simulink model "LQR_simulink"  (Simulink 7.3)
settings: Solver=ode3  StartTime=0.0  StopTime=3  FixedStep=T  RelTol=1e-3
values from neighbouring files (symbols this model uses):
  A = [0 0 0 -85.6760374833 -12.5123773517 0 0 0 0 0 -18.6077643909 -80.8140678729 ... (49 elements, 7x7)]    [A.mat]    (also in CASEfinder.m = [0 1 0; -K/m -C/m 1/m;0 0 -1/tau]; Example_check_mLyapunov.m = [0 1 0; -K/m -C/m 1/m;0 0 -1/tau]; Example_check_mriccati.m = [0 1 0; -K/m -C/m 1/m;0 0 -1/tau]; Example_in_Kang_paper.m = A_actuator)
  B = [0 0 0 0 0 62.8318530718 0 0 0 0 0 0 ... (14 elements, 7x2)]    [B.mat]    (also in CASEfinder.m = [0;0;1/tau]; Example_check_mLyapunov.m = [0;0;1/tau]; Example_check_mriccati.m = [0;0;1/tau]; Example_in_Kang_paper.m = B_actuator)
  xf = [0;0;0]    [CASEfinder.m]    (also in Main_for_DOCandDODR.m = xfn; loopsimulation.m = xf_actuator)
  xi = [0;0;0]    [CASEfinder.m]    (also in Example_check_mLyapunov.m; Example_check_mriccati.m; Main_for_DOCandDODR.m = xin; StochasticRegulator.m = zeros(7,1))
undefined symbols (not defined in the file or in its folder): Kc, T
settings Model: Creator=JSPark  LastModifiedBy=JSPark

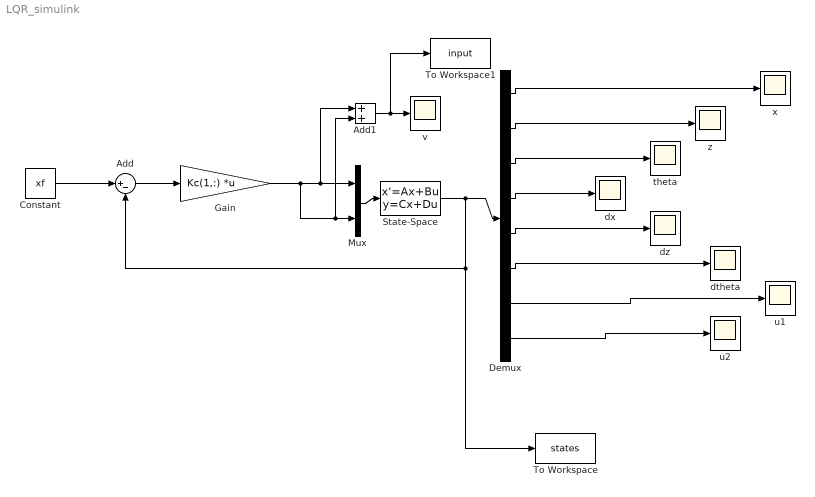
== system LQR_simulink ==
  Add : Sum  Inputs=|+-  OutDataType=fixdt(1, 16)  OutScaling=2^-10  SampleTime=T
  Add1 : Sum  OutDataType=fixdt(1, 16)  OutScaling=2^-10  SampleTime=T
  Constant : Constant  Value=xf  OutDataType=fixdt(1, 16)  OutScaling=2^0  SampleTime=T
  Demux : Demux  Outputs=8
  Gain : Gain  Gain=Kc(1,:)  Multiplication=Matrix(K*u)  ParameterDataType=fixdt(1, 16)  ParameterScaling=2^0  OutDataType=fixdt(1, 16)  OutScaling=2^0  SampleTime=T
  Mux : Mux  Inputs=2
  State-Space : StateSpace  A=A  B=B  C=eye(length(A))  D=zeros(length(A),2)  X0=xi
  To Workspace : ToWorkspace  VariableName=states  SampleTime=T  SaveFormat=Structure
  To Workspace1 : ToWorkspace  VariableName=input  SampleTime=T  SaveFormat=Structure
  dtheta : Scope
      settings: SaveName=ScopeData5
  dx : Scope
      settings: SaveName=ScopeData3
  dz : Scope
      settings: SaveName=ScopeData4
  theta : Scope
      settings: TimeRange=3  SaveName=ScopeData2
  u1 : Scope
      settings: SaveName=ScopeData6
  u2 : Scope
      settings: SaveName=ScopeData7
  v : Scope
      settings: SaveName=ScopeData8
  x : Scope
      settings: TimeRange=3
  z : Scope
  wires:
  State-Space/1 -> Demux/1, Add/2, To Workspace/1
  Add/1 -> Gain/1
  Constant/1 -> Add/1
  Mux/1 -> State-Space/1
  Gain/1 -> Mux/2, Add1/2, Mux/1, Add1/1
  Demux/1 -> x/1
  Demux/2 -> z/1
  Demux/3 -> theta/1
  Demux/4 -> dx/1
  Demux/5 -> dz/1
  Demux/6 -> dtheta/1
  Add1/1 -> v/1, To Workspace1/1
  Demux/7 -> u1/1
  Demux/8 -> u2/1
